simulink model "P_decouple_cascade_rov"  (Simulink 6.0)
settings: Solver=ode45  StartTime=0.0  StopTime=650  RelTol=1e-3
undefined symbols (not defined in the file): B, DQ, DQL, I, m, M, Ma, MaL, MaU, rg, sigbuilder_block, T, W, xb, xg, Xudot, yb, yg, Yvdot, zb, zg, Zwdot
libraries: simulink_extras x27, simulink x20
(part 2 of 5)

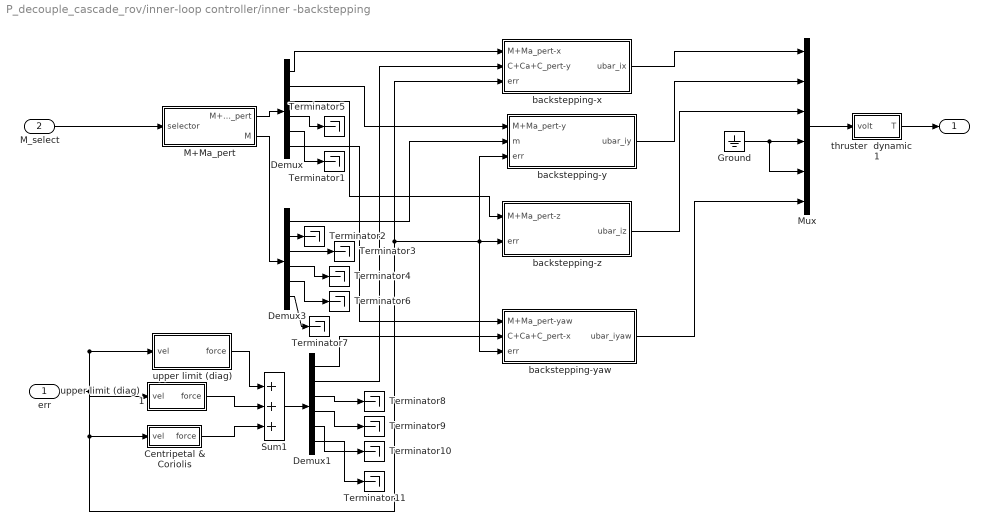
== system P_decouple_cascade_rov/inner-loop controller/inner -backstepping ==
  err : Inport  Port=1  LatchInput=off
  M_select : Inport  Port=2  LatchInput=off
  Centripetal & Coriolis : Subsystem  AncestorBlock=rov_design_analysis/ROV Models/1. Six DOF RRC ROV II/Centripetal & Coriolis
      mask Display: disp('C')
  Demux : Demux  Outputs=6
  Demux1 : Demux  Outputs=6
  Demux3 : Demux  Outputs=6
  Ground : Ground
  M+Ma_pert : Subsystem
  Mux : Mux  Inputs=6
  Sum1 : Sum  Inputs=+++  SaturateOnIntegerOverflow=on  InputSameDT=on
  Terminator{1..11} (11 alike) : Terminator
  backstepping-x : Subsystem
  backstepping-y : Subsystem
  backstepping-yaw : Subsystem
  backstepping-z : Subsystem
  thruster  dynamic     1 : Subsystem
  "upper limit (diag)   " : Subsystem
      mask Display: disp('Perturb CA')
  upper limit (diag)   1 : Subsystem
      mask Display: disp('CA')
  " " : Outport
  wires:
  M_select/1 -> M+Ma_pert/1(selector)
  err/1 -> "upper limit (diag)   "/1(vel), upper limit (diag)   1/1(vel), Centripetal & Coriolis/1(vel), backstepping-x/3(err), backstepping-y/3("err  "), backstepping-z/2("err  "), backstepping-yaw/3(err)
  M+Ma_pert/1(M+Ma_pert) -> Demux/1
  Centripetal & Coriolis/1(force) -> Sum1/3
  upper limit (diag)   1/1(force) -> Sum1/2
  "upper limit (diag)   "/1(force) -> Sum1/1
  Sum1/1 -> Demux1/1
  Demux/1 -> backstepping-x/1(M+Ma_pert-x)
  Demux1/2 -> backstepping-x/2(C+Ca+C_pert-y)
  Mux/1 -> thruster  dynamic     1/1(volt)
  M+Ma_pert/2("M ") -> Demux3/1
  Demux3/1 -> backstepping-y/2(m)
  Demux/2 -> backstepping-y/1(M+Ma_pert-y)
  Demux/6 -> backstepping-yaw/1(M+Ma_pert-yaw)
  Demux1/1 -> backstepping-yaw/2(C+Ca+C_pert-x)
  Demux/3 -> backstepping-z/1(M+Ma_pert-z)
  backstepping-x/1(ubar_ix) -> Mux/1
  backstepping-y/1(ubar_iy) -> Mux/2
  backstepping-z/1(ubar_iz) -> Mux/3
  backstepping-yaw/1(ubar_iyaw) -> Mux/6
  Ground/1 -> Mux/4, Mux/5
  Demux/4 -> Terminator5/1
  Demux/5 -> Terminator1/1
  Demux3/2 -> Terminator2/1
  Demux3/3 -> Terminator3/1
  Demux3/4 -> Terminator4/1
  Demux3/5 -> Terminator6/1
  Demux3/6 -> Terminator7/1
  Demux1/3 -> Terminator8/1
  Demux1/4 -> Terminator9/1
  Demux1/5 -> Terminator10/1
  Demux1/6 -> Terminator11/1
  thruster  dynamic     1/1(T) -> " "/1

== system P_decouple_cascade_rov/inner-loop controller/inner-P ==
  P : Inport  Port=1  LatchInput=off
  Demux1 : Demux
  Ground : Ground
  Mux2 : Mux  Inputs=6
  P Controller{1..4} (4 alike) : simulink_extras/Additional Linear/PID Controller  P=1  I=0  D=0
  Selector : Selector  Elements=[1 2 3 6]  InputPortWidth=6
  thruster  dynamic     1 : Subsystem
  " " : Outport
  wires:
  P Controller3/1 -> Mux2/3
  P Controller1/1 -> Mux2/1
  P Controller2/1 -> Mux2/2
  Selector/1 -> Demux1/1
  Demux1/1 -> P Controller1/1
  Demux1/2 -> P Controller2/1
  Demux1/3 -> P Controller3/1
  Demux1/4 -> P Controller4/1
  P Controller4/1 -> Mux2/6
  Ground/1 -> Mux2/4, Mux2/5
  P/1 -> Selector/1
  Mux2/1 -> thruster  dynamic     1/1(volt)
  thruster  dynamic     1/1(T) -> " "/1

== system P_decouple_cascade_rov/inner-loop controller/inner-sliding ==
  sliding : Inport  Port=1  LatchInput=off
  Sign : Signum
  thruster  dynamic     1 : Subsystem
  " " : Outport
  wires:
  Sign/1 -> thruster  dynamic     1/1(volt)
  sliding/1 -> Sign/1
  thruster  dynamic     1/1(T) -> " "/1

== system P_decouple_cascade_rov/outer-loop  controller/P ==
  err : Inport  Port=1  LatchInput=off
  Demux1 : Demux  Outputs=6
  Mux2 : Mux  Inputs=6
  P Controller{1..4} (4 alike) : simulink_extras/Additional Linear/PID Controller  P=1  I=0  D=0
  " " : Outport
  wires:
  P Controller3/1 -> Mux2/3
  err/1 -> Demux1/1
  Mux2/1 -> " "/1
  Demux1/1 -> P Controller1/1
  P Controller1/1 -> Mux2/1
  P Controller2/1 -> Mux2/2
  P Controller4/1 -> Mux2/6
  Demux1/2 -> P Controller2/1
  Demux1/3 -> P Controller3/1
  Demux1/6 -> P Controller4/1

== system P_decouple_cascade_rov/outer-loop  controller/PI sine +nonlinear  ==
  err : Inport  Port=1  LatchInput=off
  Demux1 : Demux  Outputs=6
  Mux2 : Mux  Inputs=6
  P Controller1 : simulink_extras/Additional Linear/PID Controller  P=1  I=1  D=0
  P Controller2 : simulink_extras/Additional Linear/PID Controller  P=1  I=1  D=0
  P Controller3 : simulink_extras/Additional Linear/PID Controller  P=1  I=1  D=0
  Subsystem : Subsystem
  " " : Outport
  wires:
  P Controller3/1 -> Mux2/3
  err/1 -> Demux1/1
  Mux2/1 -> " "/1
  Demux1/1 -> Subsystem/1(xe), P Controller1/1
  P Controller1/1 -> Mux2/1
  P Controller2/1 -> Mux2/2
  Subsystem/1(yaw_angle) -> Mux2/6
  Demux1/2 -> P Controller2/1, Subsystem/2(ye)
  Demux1/3 -> P Controller3/1

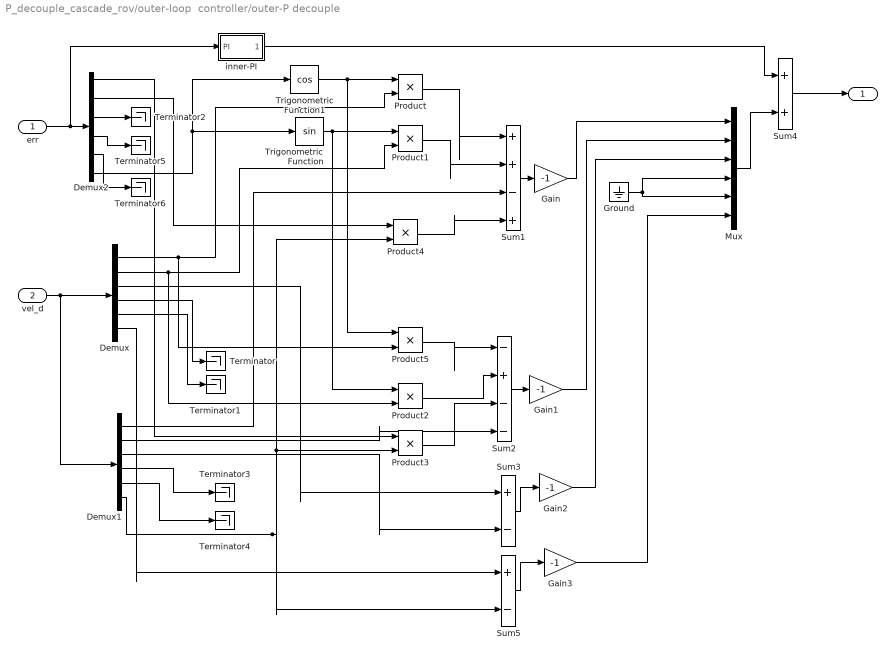
== system P_decouple_cascade_rov/outer-loop  controller/outer-P decouple  ==
  err : Inport  Port=1  LatchInput=off
  vel_d : Inport  Port=2  LatchInput=off
  Demux : Demux  Outputs=6
  Demux1 : Demux  Outputs=6
  Demux2 : Demux  Outputs=6
  Gain{,1..3} (4 alike) : Gain  Gain=-1
  Ground : Ground
  Mux : Mux  Inputs=6
  Product{,1..4} (5 alike) : Product  RndMeth=Zero
  Product5 : Product  OutDataTypeMode=double  RndMeth=Zero
  Sum1 : Sum  Inputs=|++-+  SaturateOnIntegerOverflow=on  InputSameDT=on
  Sum2 : Sum  Inputs=|-+--  SaturateOnIntegerOverflow=on  InputSameDT=on
  Sum3 : Sum  Inputs=|+-  SaturateOnIntegerOverflow=on  InputSameDT=on
  Sum4 : Sum  Inputs=|++  SaturateOnIntegerOverflow=on  InputSameDT=on
  Sum5 : Sum  Inputs=|+-  SaturateOnIntegerOverflow=on  InputSameDT=on
  Terminator{,1..6} (7 alike) : Terminator
  Trigonometric Function : Trigonometry
  Trigonometric Function1 : Trigonometry  Operator=cos
  inner-PI : Subsystem
  " " : Outport
  wires:
  err/1 -> Demux2/1, inner-PI/1(PI)
  vel_d/1 -> Demux/1, Demux1/1
  Sum2/1 -> Gain1/1
  Sum1/1 -> Gain/1
  Sum3/1 -> Gain2/1
  Ground/1 -> Mux/4, Mux/5
  Demux1/4 -> Terminator3/1
  Demux1/5 -> Terminator4/1
  Trigonometric Function/1 -> Product1/1, Product2/1
  Trigonometric Function1/1 -> Product/1, Product5/1
  Demux2/6 -> Trigonometric Function1/1, Trigonometric Function/1
  Demux/1 -> Product5/2, Product/2
  Demux/2 -> Product2/2, Product1/2
  Product/1 -> Sum1/1
  Product1/1 -> Sum1/2
  Demux1/1 -> Sum1/3
  Product4/1 -> Sum1/4
  Demux1/6 -> Product4/2, Product3/2, Sum5/2
  Demux2/2 -> Product4/1
  Product5/1 -> Sum2/1
  Product2/1 -> Sum2/2
  Product3/1 -> Sum2/3
  Demux2/1 -> Product3/1
  Demux1/2 -> Sum2/4
  Demux/3 -> Sum3/1
  Demux1/3 -> Sum3/2
  Demux/4 -> Terminator/1
  Demux/5 -> Terminator1/1
  Gain/1 -> Mux/1
  Gain1/1 -> Mux/2
  Gain2/1 -> Mux/3
  inner-PI/1(" ") -> Sum4/1
  Mux/1 -> Sum4/2
  Sum4/1 -> " "/1
  Demux2/3 -> Terminator2/1
  Demux2/4 -> Terminator5/1
  Demux2/5 -> Terminator6/1
  Demux/6 -> Sum5/1
  Sum5/1 -> Gain3/1
  Gain3/1 -> Mux/6

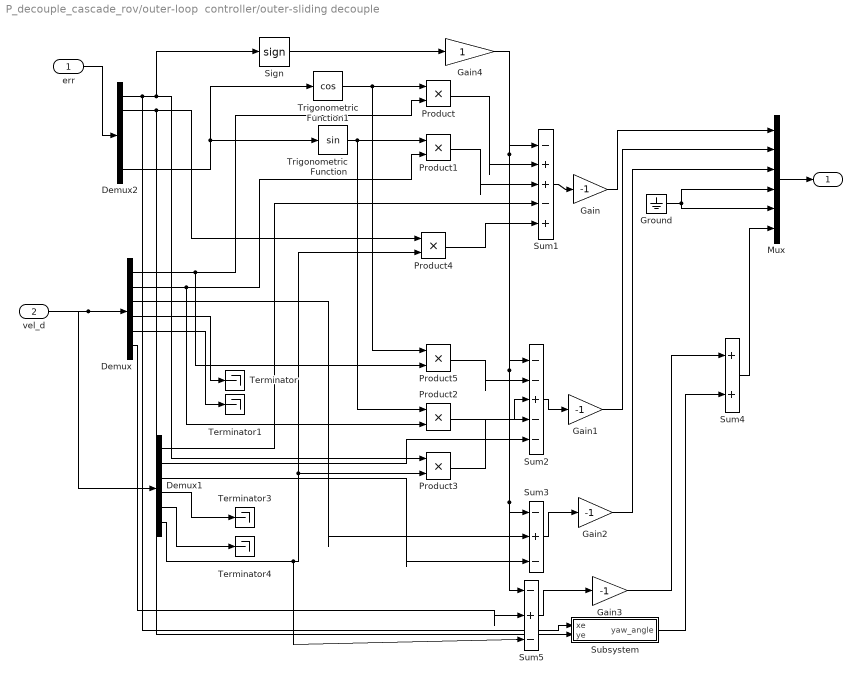
== system P_decouple_cascade_rov/outer-loop  controller/outer-sliding decouple ==
  err : Inport  Port=1  LatchInput=off
  vel_d : Inport  Port=2  LatchInput=off
  Demux : Demux  Outputs=6
  Demux1 : Demux  Outputs=6
  Demux2 : Demux  Outputs=6
  Gain{,1..3} (4 alike) : Gain  Gain=-1
  Gain4 : Gain  SaturateOnIntegerOverflow=on
  Ground : Ground
  Mux : Mux  Inputs=6
  Product{,1..4} (5 alike) : Product  RndMeth=Zero
  Product5 : Product  OutDataTypeMode=double  RndMeth=Zero
  Sign : Signum
  Subsystem : Subsystem
  Sum1 : Sum  Inputs=|-++-+  SaturateOnIntegerOverflow=on  InputSameDT=on
  Sum2 : Sum  Inputs=|--+--  SaturateOnIntegerOverflow=on  InputSameDT=on
  Sum3 : Sum  Inputs=|-+-  SaturateOnIntegerOverflow=on  InputSameDT=on
  Sum4 : Sum  Inputs=|++  SaturateOnIntegerOverflow=on  InputSameDT=on
  Sum5 : Sum  Inputs=|-+-  SaturateOnIntegerOverflow=on  InputSameDT=on
  Terminator{,1,3..4} (4 alike) : Terminator
  Trigonometric Function : Trigonometry
  Trigonometric Function1 : Trigonometry  Operator=cos
  " " : Outport
  wires:
  err/1 -> Demux2/1
  vel_d/1 -> Demux/1, Demux1/1
  Sum2/1 -> Gain1/1
  Sum1/1 -> Gain/1
  Sum3/1 -> Gain2/1
  Sum5/1 -> Gain3/1
  Ground/1 -> Mux/4, Mux/5
  Demux1/4 -> Terminator3/1
  Demux1/5 -> Terminator4/1
  Trigonometric Function/1 -> Product1/1, Product2/1
  Trigonometric Function1/1 -> Product/1, Product5/1
  Demux2/6 -> Trigonometric Function1/1, Trigonometric Function/1
  Demux/1 -> Product/2, Product5/2
  Demux/2 -> Product1/2, Product2/2
  Product/1 -> Sum1/2
  Product1/1 -> Sum1/3
  Demux1/1 -> Sum1/4
  Product4/1 -> Sum1/5
  Demux1/6 -> Product4/2, Product3/2, Sum5/3
  Demux2/2 -> Product4/1, Subsystem/2(ye)
  Product5/1 -> Sum2/2
  Product2/1 -> Sum2/3
  Product3/1 -> Sum2/4
  Demux2/1 -> Product3/1, Sign/1, Subsystem/1(xe)
  Demux1/2 -> Sum2/5
  Demux/3 -> Sum3/2
  Demux1/3 -> Sum3/3
  Demux/6 -> Sum5/2
  Demux/4 -> Terminator/1
  Demux/5 -> Terminator1/1
  Gain/1 -> Mux/1
  Gain1/1 -> Mux/2
  Gain2/1 -> Mux/3
  Sign/1 -> Gain4/1
  Mux/1 -> " "/1
  Gain4/1 -> Sum1/1, Sum2/1, Sum3/1, Sum5/1
  Gain3/1 -> Sum4/1
  Subsystem/1(yaw_angle) -> Sum4/2
  Sum4/1 -> Mux/6

== system P_decouple_cascade_rov/pipeline  tracking planner  /decoupled input ==
  In1 : Inport  Orientation=down  Port=1  LatchInput=off
  relative pt : MultiPortSwitch  Inputs=8
  "x25, y=0, z=50 yaw=1.57" : Subsystem
  "x=0,y=0, z=0 yaw=0  " : Subsystem
  "x=15,y=0, z=45 yaw=0 " : Subsystem
  "x=25, z=45 yaw=0" : Subsystem
  "x=25,y=0, z=50 yaw=0" : Subsystem
  "x=25,y=40, z=50 yaw=0" : Subsystem
  "x=y=0, z=-50 yaw=0  " : Subsystem
  "x=y=15, z=50 yaw=0 " : Subsystem
  Out1 : Outport
  wires:
  "x=y=0, z=-50 yaw=0  "/1("1 ") -> relative pt/2  "1"
  "x=y=15, z=50 yaw=0 "/1(2) -> relative pt/3  "2"
  "x=15,y=0, z=45 yaw=0 "/1(3) -> relative pt/4  "3"
  "x=25, z=45 yaw=0"/1(4) -> relative pt/5  "4"
  "x=25,y=0, z=50 yaw=0"/1(5) -> relative pt/6  "5"
  "x25, y=0, z=50 yaw=1.57"/1(6) -> relative pt/7  "6"
  "x=25,y=40, z=50 yaw=0"/1(7) -> relative pt/8  "7"
  "x=0,y=0, z=0 yaw=0  "/1(8) -> relative pt/9  "8"
  In1/1 -> relative pt/1
  relative pt/1 -> Out1/1

== system P_decouple_cascade_rov/(Observer/ Six DOF RRC ROV   1/Centripetal & Coriolis ==
  vel : Inport  Orientation=up  Port=1  LatchInput=off
  Demux : Demux  Orientation=up  Outputs=2
  Mux : Mux  Inputs=2
  Product{1..5} (5 alike) : Product  SaturateOnIntegerOverflow=on  RndMeth=Zero  InputSameDT=on
  Rg : Constant  Value=rg
  Sum : Sum  SaturateOnIntegerOverflow=on  InputSameDT=on
  Sum1 : Sum  SaturateOnIntegerOverflow=on  InputSameDT=on
  inertia(3x3) : Gain  Gain=I*eye(3)+[Xudot 0 0;0 Yvdot 0;0 0 Zwdot]  Multiplication=Matrix(K*u)  SaturateOnIntegerOverflow=on
  "mass(3x3) " : Gain  Gain=m*eye(3)+[Xudot 0 0;0 Yvdot 0;0 0 Zwdot]  Multiplication=Matrix(K*u)  SaturateOnIntegerOverflow=on
  "mass(3x3)   " : Gain  Gain=m*eye(3)+[Xudot 0 0;0 Yvdot 0;0 0 Zwdot]  Multiplication=Matrix(K*u)  SaturateOnIntegerOverflow=on
  force : Outport  InitialOutput=0
  wires:
  Product1/1 -> Sum/2
  "mass(3x3)   "/1 -> Product2/1
  Product2/1 -> Sum/1
  Rg/1 -> Product3/2, "mass(3x3)   "/1
  Product3/1 -> Product4/2
  Product4/1 -> Sum1/1
  Product5/1 -> Product2/2, Sum1/2
  Sum1/1 -> "mass(3x3) "/1
  Demux/2 -> Product5/1, Product3/1, Product4/1, Product1/1, inertia(3x3)/1
  Demux/1 -> Product5/2
  vel/1 -> Demux/1
  inertia(3x3)/1 -> Product1/2
  "mass(3x3) "/1 -> Mux/1
  Sum/1 -> Mux/2
  Mux/1 -> force/1

== system P_decouple_cascade_rov/(Observer/ Six DOF RRC ROV   1/Hydrodynamic  Damping ==
  vel : Inport  Port=1  LatchInput=off
  D linear : Gain  Gain=-diag(DQL)  SaturateOnIntegerOverflow=on
  damping force : Outport  InitialOutput=0
  wires:
  vel/1 -> D linear/1
  D linear/1 -> damping force/1

== system P_decouple_cascade_rov/(Observer/ Six DOF RRC ROV   1/Hydrodynamic  Damping1 ==
  vel : Inport  Port=1  LatchInput=off
  D quadratic : Gain  Gain=-diag(DQ)  SaturateOnIntegerOverflow=on
  Product : Product  SaturateOnIntegerOverflow=on  RndMeth=Zero  InputSameDT=on
  |u| : Abs  SaturateOnIntegerOverflow=on
  damping force : Outport  InitialOutput=0
  wires:
  Product/1 -> D quadratic/1
  vel/1 -> Product/1, |u|/1
  |u|/1 -> Product/2
  D quadratic/1 -> damping force/1

== system P_decouple_cascade_rov/(Observer/ Six DOF RRC ROV   1/Hydrodynamic  Damping2 ==
  vel : Inport  Port=1  LatchInput=off
  D quadratic : Gain  Gain=0  SaturateOnIntegerOverflow=on
  damping force : Outport  InitialOutput=0
  wires:
  D quadratic/1 -> damping force/1
  vel/1 -> D quadratic/1

== system P_decouple_cascade_rov/(Observer/ Six DOF RRC ROV   1/Mass Inertia Matrix ==
  In : Inport  Port=1  LatchInput=off
  inverse M : Gain  Gain=inv(M-Ma)  Multiplication=Matrix(K*u)  SaturateOnIntegerOverflow=on
  Out : Outport
  wires:
  inverse M/1 -> Out/1
  In/1 -> inverse M/1

== system P_decouple_cascade_rov/(Observer/ Six DOF RRC ROV   1/Restoring Forces ==
  pos : Inport  Port=1  LatchInput=off
  (xg.W-xb.B)cY.cX : Fcn  Expr=(xg*W - xb*B)*cos(u[2])*cos(u[1])
  (zg.W - zb.B)cY.sX : Fcn  Expr=((zg * W - zb * B) * cos(u[2])) * sin(u[1])
  (zg.W - zb.B)sY : Fcn  Expr=(zg*W - zb*B)*sin(u[2])
  -(xg.W-xb.B)cY.sX : Fcn  Expr=-(xg*W - xb*B)*cos(u[2])*sin(u[1])
  -(yg.W-yb.B)cY.cX : Fcn  Expr=-(yg*W - yb*B)*cos(u[2])*cos(u[1])
  -(yg.W-yb.B)sY : Fcn  Expr=-(yg*W - yb*B)*sin(u[2])
  -cY.cX : Fcn  Expr=-cos(u[2])*cos(u[1])
  -cY.sX : Fcn  Expr=-cos(u[2])*sin(u[1])
  Demux : Demux  Outputs=2
  Gain : Gain  Gain=W-B  SaturateOnIntegerOverflow=on
  Mux : Mux  Inputs=3
  Mux1 : Mux
  Sum : Sum  SaturateOnIntegerOverflow=on  InputSameDT=on
  Sum1 : Sum  SaturateOnIntegerOverflow=on  InputSameDT=on
  Sum2 : Sum  SaturateOnIntegerOverflow=on  InputSameDT=on
  Terminator : Terminator
  sY : Fcn  Expr=sin(u[2])
  gravitational force : Outport  InitialOutput=0
  wires:
  Sum2/1 -> Mux1/4
  -(yg.W-yb.B)sY/1 -> Sum2/1
  -(xg.W-xb.B)cY.sX/1 -> Sum2/2
  Sum1/1 -> Mux1/3
  (xg.W-xb.B)cY.cX/1 -> Sum1/1
  (zg.W - zb.B)sY/1 -> Sum1/2
  Sum/1 -> Mux1/2
  (zg.W - zb.B)cY.sX/1 -> Sum/1
  -(yg.W-yb.B)cY.cX/1 -> Sum/2
  Gain/1 -> Mux1/1
  Mux/1 -> Gain/1
  -cY.cX/1 -> Mux/3
  -cY.sX/1 -> Mux/2
  sY/1 -> Mux/1
  Mux1/1 -> gravitational force/1
  Demux/2 -> -(xg.W-xb.B)cY.sX/1, -(yg.W-yb.B)sY/1, (zg.W - zb.B)sY/1, (xg.W-xb.B)cY.cX/1, -(yg.W-yb.B)cY.cX/1, (zg.W - zb.B)cY.sX/1, sY/1, -cY.sX/1, -cY.cX/1
  Demux/1 -> Terminator/1
  pos/1 -> Demux/1

== system P_decouple_cascade_rov/(Observer/ Six DOF RRC ROV   1/lower limit (diag) ==
  In : Inport  Port=1  LatchInput=off
  inverse M : Gain  Gain=-diag([21.1403-21.0981 51.7012-51.0026 92.451-91.837 3.6191-3.576 2.6427-2.7687 2.3033-2.3493])  Multiplication=Matrix(K*u)  SaturateOnIntegerOverflow=on
  Out : Outport
  wires:
  inverse M/1 -> Out/1
  In/1 -> inverse M/1

== system P_decouple_cascade_rov/(Observer/ Six DOF RRC ROV   1/upper limit (diag) ==
  In : Inport  Port=1  LatchInput=off
  inverse M : Gain  Gain=-diag([21.724-21.1403 51.7013-51.7012 94.3-92.451 4.2176-3.6191 7.1148-2.6427 4.7673-2.3033])  Multiplication=Matrix(K*u)  SaturateOnIntegerOverflow=on
  Out : Outport
  wires:
  inverse M/1 -> Out/1
  In/1 -> inverse M/1

== system P_decouple_cascade_rov/(Observer/ Six DOF RRC ROV   1/upper limit (diag)    ==
  note: 7 8 9 10 11 12
  note: 1 2 3 4 5 6
  vel : Inport  Port=1  LatchInput=off
  (zg.W - zb.B)cY.sX : Fcn  Expr=-u[9]*u[3]*u[5]+u[8]*u[2]*u[6]
  (zg.W - zb.B)cY.sX1 : Fcn  Expr=u[9]*u[3]*u[4]-u[7]*u[1]*u[6]
  (zg.W - zb.B)cY.sX2 : Fcn  Expr=-u[8]*u[2]*u[4]+u[7]*u[1]*u[5]
  (zg.W - zb.B)cY.sX3 : Fcn  Expr=-u[9]*u[3]*u[2]+u[8]*u[2]*u[3]-u[12]*u[6]*u[5]+u[11]*u[5]*u[6]
  (zg.W - zb.B)cY.sX4 : Fcn  Expr=u[9]*u[3]*u[1]-u[7]*u[1]*u[3]+u[6]*u[12]*u[4]-u[4]*u[10]*u[6]
  (zg.W - zb.B)cY.sX5 : Fcn  Expr=-u[8]*u[2]*u[1]+u[7]*u[1]*u[2]-u[11]*u[5]*u[4]+u[10]*u[4]*u[5]
  Mux1 : Mux  Inputs=6
  Mux3 : Mux  Inputs=2
  Rg1 : Constant  Value="[MaU(1)  MaU(2)  MaU(3)  MaU(4)  MaU(5)  MaU(6) ]'"
  force : Outport
  wires:
  Mux1/1 -> force/1
  (zg.W - zb.B)cY.sX/1 -> Mux1/1
  (zg.W - zb.B)cY.sX1/1 -> Mux1/2
  (zg.W - zb.B)cY.sX2/1 -> Mux1/3
  (zg.W - zb.B)cY.sX3/1 -> Mux1/4
  (zg.W - zb.B)cY.sX4/1 -> Mux1/5
  (zg.W - zb.B)cY.sX5/1 -> Mux1/6
  vel/1 -> Mux3/1
  Rg1/1 -> Mux3/2
  Mux3/1 -> (zg.W - zb.B)cY.sX/1, (zg.W - zb.B)cY.sX1/1, (zg.W - zb.B)cY.sX4/1, (zg.W - zb.B)cY.sX5/1, (zg.W - zb.B)cY.sX3/1, (zg.W - zb.B)cY.sX2/1

== system P_decouple_cascade_rov/(Observer/ Six DOF RRC ROV   1/upper limit (diag)   1 ==
  note: 7 8 9 10 11 12
  note: 1 2 3 4 5 6
  vel : Inport  Port=1  LatchInput=off
  (zg.W - zb.B)cY.sX : Fcn  Expr=-u[9]*u[3]*u[5]+u[8]*u[2]*u[6]
  (zg.W - zb.B)cY.sX1 : Fcn  Expr=u[9]*u[3]*u[4]-u[7]*u[1]*u[6]
  (zg.W - zb.B)cY.sX2 : Fcn  Expr=-u[8]*u[2]*u[4]+u[7]*u[1]*u[5]
  (zg.W - zb.B)cY.sX3 : Fcn  Expr=-u[9]*u[3]*u[2]+u[8]*u[2]*u[3]-u[12]*u[6]*u[5]+u[11]*u[5]*u[6]
  (zg.W - zb.B)cY.sX4 : Fcn  Expr=u[9]*u[3]*u[1]-u[7]*u[1]*u[3]+u[6]*u[12]*u[4]-u[4]*u[10]*u[6]
  (zg.W - zb.B)cY.sX5 : Fcn  Expr=-u[8]*u[2]*u[1]+u[7]*u[1]*u[2]-u[11]*u[5]*u[4]+u[10]*u[4]*u[5]
  Mux1 : Mux  Inputs=6
  Mux3 : Mux  Inputs=2
  Rg1 : Constant  Value="[Ma(1)  Ma(2)  Ma(3)  Ma(4)  Ma(5)  Ma(6) ]'"
  force : Outport
  wires:
  Mux1/1 -> force/1
  (zg.W - zb.B)cY.sX/1 -> Mux1/1
  (zg.W - zb.B)cY.sX1/1 -> Mux1/2
  (zg.W - zb.B)cY.sX2/1 -> Mux1/3
  (zg.W - zb.B)cY.sX3/1 -> Mux1/4
  (zg.W - zb.B)cY.sX4/1 -> Mux1/5
  (zg.W - zb.B)cY.sX5/1 -> Mux1/6
  vel/1 -> Mux3/1
  Rg1/1 -> Mux3/2
  Mux3/1 -> (zg.W - zb.B)cY.sX/1, (zg.W - zb.B)cY.sX1/1, (zg.W - zb.B)cY.sX4/1, (zg.W - zb.B)cY.sX5/1, (zg.W - zb.B)cY.sX3/1, (zg.W - zb.B)cY.sX2/1

== system P_decouple_cascade_rov/(Observer/ Six DOF RRC ROV   1/upper limit1 ==
  In : Inport  Port=1  LatchInput=off
  inverse M : Gain  Gain=0  Multiplication=Matrix(K*u)  SaturateOnIntegerOverflow=on
  Out : Outport
  wires:
  inverse M/1 -> Out/1
  In/1 -> inverse M/1

== system P_decouple_cascade_rov/(Observer/Euler  Transformation1/Transformation matrix R ==
  angular body  velocity : Inport  Port=1  LatchInput=off
  angular position : Inport  Port=2  LatchInput=off
  Mux : Mux  Inputs=3
  Row1 of T : Subsystem
      mask Display: disp('Row 1')
  Row2 of T : Subsystem
      mask Display: disp('Row 2')
  Row3 of T : Subsystem
      mask Display: disp('Row 3')
  angular earth velocity : Outport
  wires:
  angular position/1 -> Row3 of T/2(angular position), Row1 of T/2(angular position), Row2 of T/2(angular position)
  Mux/1 -> angular earth velocity/1
  Row3 of T/1(angular earth velocity (row 3)) -> Mux/3
  Row2 of T/1(angular earth velocity (row 2)) -> Mux/2
  Row1 of T/1(angular earth velocity (row 1)) -> Mux/1
  angular body  velocity/1 -> Row3 of T/1("angular body velocity "), Row2 of T/1("angular body velocity "), Row1 of T/1(angular body  velocity)

== system P_decouple_cascade_rov/(Observer/Euler  Transformation1/Transformation matrix T ==
  translational body velocity : Inport  Port=1  LatchInput=off
  angular position : Inport  Port=2  LatchInput=off
  Mux : Mux  Inputs=3
  Row1 of R : Subsystem
      mask Display: disp('Row 1')
  Row2 of R : Subsystem
      mask Display: disp('Row 2')
  Row3 of R : Subsystem
      mask Display: disp('Row 3')
  translational earth velocity : Outport  InitialOutput=0
  wires:
  Mux/1 -> translational earth velocity/1
  Row3 of R/1(translational earth velocity (row 3)) -> Mux/3
  Row2 of R/1(translational earth velocity (row 2)) -> Mux/2
  Row1 of R/1(translational earth velocity (row 1)) -> Mux/1
  angular position/1 -> Row3 of R/2(angular position), Row1 of R/2(angular position), Row2 of R/2(angular position)
  translational body velocity/1 -> Row1 of R/1(translational body velocity), Row2 of R/1(translational body velocity), Row3 of R/1(translational body velocity)

== system P_decouple_cascade_rov/(Observer/Thruster  Dynamic/Thruster configuration1 ==
  input velocity : Inport  Orientation=up  Port=1  LatchInput=off
  Thruster Matrix : Gain  Gain=T  Multiplication=Matrix(K*u)  SaturateOnIntegerOverflow=on
  output force : Outport  InitialOutput=0
  wires:
  input velocity/1 -> Thruster Matrix/1
  Thruster Matrix/1 -> output force/1

== system P_decouple_cascade_rov/(Observer/Thruster  Dynamic/Thruster configuration4 ==
  input velocity : Inport  Orientation=up  Port=1  LatchInput=off
  Thruster Matrix : Gain  Gain=T  Multiplication=Matrix(K*u)  SaturateOnIntegerOverflow=on
  output force : Outport  InitialOutput=0
  wires:
  input velocity/1 -> Thruster Matrix/1
  Thruster Matrix/1 -> output force/1

== system P_decouple_cascade_rov/(Observer/Thruster  Dynamic/thruster  dynamic     1 ==
  volt : Inport  Orientation=down  Port=1  LatchInput=off
  Gain2 : Gain  Gain=0.5  SaturateOnIntegerOverflow=on
  Saturation : Saturate  UpperLimit=70  LowerLimit=-70
  "thruster  alloc. " : Subsystem
  T : Outport
  wires:
  volt/1 -> "thruster  alloc. "/1(err)
  "thruster  alloc. "/1(u) -> Gain2/1
  Saturation/1 -> T/1
  Gain2/1 -> Saturation/1

== system P_decouple_cascade_rov/(Observer/inner-loop controller1/inner -PI-decouple  ==
  err : Inport  Port=1  LatchInput=off
  Centripetal & Coriolis : Subsystem  AncestorBlock=rov_design_analysis/ROV Models/1. Six DOF RRC ROV II/Centripetal & Coriolis
      mask Display: disp('C')
  Gain2 : Gain  SaturateOnIntegerOverflow=on
  Hydrodynamic  Damping : Subsystem
      mask Display: disp('D')
  Hydrodynamic  Damping1 : Subsystem
      mask Display: disp('Perturb D')
  Sum : Sum  Inputs=|-++  SaturateOnIntegerOverflow=on  InputSameDT=on
  Sum1 : Sum  Inputs=+++  SaturateOnIntegerOverflow=on  InputSameDT=on
  Sum5 : Sum  Inputs=|++  SaturateOnIntegerOverflow=on  InputSameDT=on
  inner-PI : Subsystem
  thruster  dynamic     1 : Subsystem
  "upper limit (diag)   " : Subsystem
      mask Display: disp('Perturb CA')
  upper limit (diag)   1 : Subsystem
      mask Display: disp('CA')
  " " : Outport
  wires:
  err/1 -> upper limit (diag)   1/1(vel), Centripetal & Coriolis/1(vel), "upper limit (diag)   "/1(vel), Hydrodynamic  Damping/1(vel), Hydrodynamic  Damping1/1(vel), inner-PI/1(PI)
  upper limit (diag)   1/1(force) -> Sum1/1
  Centripetal & Coriolis/1(force) -> Sum1/2
  Hydrodynamic  Damping1/1(damping force) -> Sum5/2
  inner-PI/1(" ") -> Gain2/1
  "upper limit (diag)   "/1(force) -> Sum1/3
  Hydrodynamic  Damping/1(damping force) -> Sum5/1
  Gain2/1 -> Sum/1
  Sum5/1 -> Sum/3
  Sum1/1 -> Sum/2
  Sum/1 -> thruster  dynamic     1/1(volt)
  thruster  dynamic     1/1(T) -> " "/1

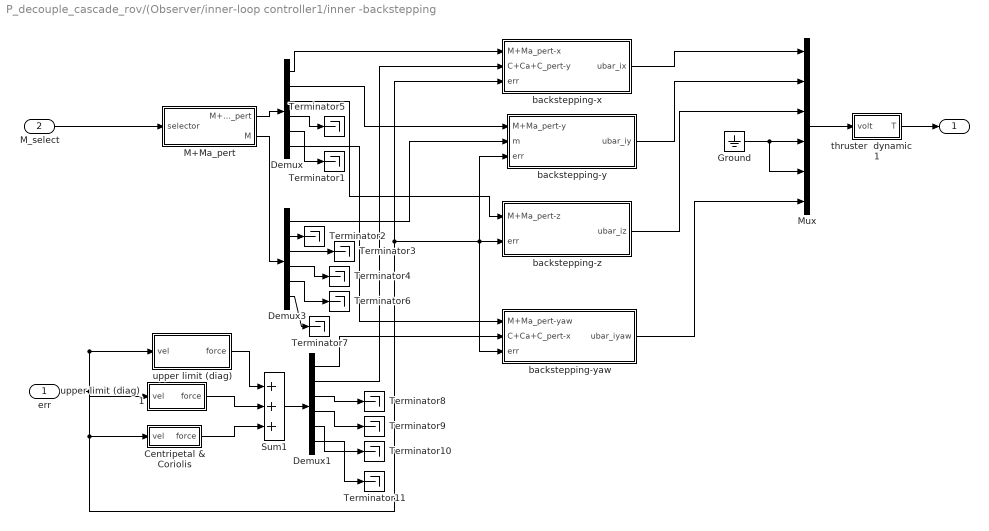
== system P_decouple_cascade_rov/(Observer/inner-loop controller1/inner -backstepping ==
  err : Inport  Port=1  LatchInput=off
  M_select : Inport  Port=2  LatchInput=off
  Centripetal & Coriolis : Subsystem  AncestorBlock=rov_design_analysis/ROV Models/1. Six DOF RRC ROV II/Centripetal & Coriolis
      mask Display: disp('C')
  Demux : Demux  Outputs=6
  Demux1 : Demux  Outputs=6
  Demux3 : Demux  Outputs=6
  Ground : Ground
  M+Ma_pert : Subsystem
  Mux : Mux  Inputs=6
  Sum1 : Sum  Inputs=+++  SaturateOnIntegerOverflow=on  InputSameDT=on
  Terminator{1..11} (11 alike) : Terminator
  backstepping-x : Subsystem
  backstepping-y : Subsystem
  backstepping-yaw : Subsystem
  backstepping-z : Subsystem
  thruster  dynamic     1 : Subsystem
  "upper limit (diag)   " : Subsystem
      mask Display: disp('Perturb CA')
  upper limit (diag)   1 : Subsystem
      mask Display: disp('CA')
  " " : Outport
  wires:
  M_select/1 -> M+Ma_pert/1(selector)
  err/1 -> "upper limit (diag)   "/1(vel), upper limit (diag)   1/1(vel), Centripetal & Coriolis/1(vel), backstepping-x/3(err), backstepping-y/3("err  "), backstepping-z/2("err  "), backstepping-yaw/3(err)
  M+Ma_pert/1(M+Ma_pert) -> Demux/1
  Centripetal & Coriolis/1(force) -> Sum1/3
  upper limit (diag)   1/1(force) -> Sum1/2
  "upper limit (diag)   "/1(force) -> Sum1/1
  Sum1/1 -> Demux1/1
  Demux/1 -> backstepping-x/1(M+Ma_pert-x)
  Demux1/2 -> backstepping-x/2(C+Ca+C_pert-y)
  Mux/1 -> thruster  dynamic     1/1(volt)
  M+Ma_pert/2("M ") -> Demux3/1
  Demux3/1 -> backstepping-y/2(m)
  Demux/2 -> backstepping-y/1(M+Ma_pert-y)
  Demux/6 -> backstepping-yaw/1(M+Ma_pert-yaw)
  Demux1/1 -> backstepping-yaw/2(C+Ca+C_pert-x)
  Demux/3 -> backstepping-z/1(M+Ma_pert-z)
  backstepping-x/1(ubar_ix) -> Mux/1
  backstepping-y/1(ubar_iy) -> Mux/2
  backstepping-z/1(ubar_iz) -> Mux/3
  backstepping-yaw/1(ubar_iyaw) -> Mux/6
  Ground/1 -> Mux/4, Mux/5
  Demux/4 -> Terminator5/1
  Demux/5 -> Terminator1/1
  Demux3/2 -> Terminator2/1
  Demux3/3 -> Terminator3/1
  Demux3/4 -> Terminator4/1
  Demux3/5 -> Terminator6/1
  Demux3/6 -> Terminator7/1
  Demux1/3 -> Terminator8/1
  Demux1/4 -> Terminator9/1
  Demux1/5 -> Terminator10/1
  Demux1/6 -> Terminator11/1
  thruster  dynamic     1/1(T) -> " "/1

== system P_decouple_cascade_rov/(Observer/inner-loop controller1/inner-P ==
  P : Inport  Port=1  LatchInput=off
  Demux1 : Demux
  Ground : Ground
  Mux2 : Mux  Inputs=6
  P Controller{1..4} (4 alike) : simulink_extras/Additional Linear/PID Controller  P=1  I=0  D=0
  Selector : Selector  Elements=[1 2 3 6]  InputPortWidth=6
  thruster  dynamic     1 : Subsystem
  " " : Outport
  wires:
  P Controller3/1 -> Mux2/3
  P Controller1/1 -> Mux2/1
  P Controller2/1 -> Mux2/2
  Selector/1 -> Demux1/1
  Demux1/1 -> P Controller1/1
  Demux1/2 -> P Controller2/1
  Demux1/3 -> P Controller3/1
  Demux1/4 -> P Controller4/1
  P Controller4/1 -> Mux2/6
  Ground/1 -> Mux2/4, Mux2/5
  P/1 -> Selector/1
  Mux2/1 -> thruster  dynamic     1/1(volt)
  thruster  dynamic     1/1(T) -> " "/1

== system P_decouple_cascade_rov/(Observer/inner-loop controller1/inner-sliding ==
  sliding : Inport  Port=1  LatchInput=off
  Sign : Signum
  thruster  dynamic     1 : Subsystem
  " " : Outport
  wires:
  Sign/1 -> thruster  dynamic     1/1(volt)
  sliding/1 -> Sign/1
  thruster  dynamic     1/1(T) -> " "/1

== system P_decouple_cascade_rov/Euler  Transformation/Transformation matrix R/Row1 of T ==
  angular body  velocity : Inport  Port=1  LatchInput=off
  angular position : Inport  Port=2  LatchInput=off
  1 : Fcn  Expr=1
  Dot Product1 : simulink/Math Operations/Dot Product  InputSameDT=on  OutDataType=sfix(16)  OutScaling=2^-10  DoSatur=off
  Mux1 : Mux  Inputs=3
  cX.tY : Fcn  Expr=cos(u[1])*tan(u[2])
  sX.tY : Fcn  Expr=sin(u[1])*tan(u[2])
  angular earth velocity (row 1) : Outport
  wires:
  Dot Product1/1 -> angular earth velocity (row 1)/1
  angular body  velocity/1 -> Dot Product1/2
  Mux1/1 -> Dot Product1/1
  cX.tY/1 -> Mux1/3
  sX.tY/1 -> Mux1/2
  1/1 -> Mux1/1
  angular position/1 -> cX.tY/1, sX.tY/1, 1/1

== system P_decouple_cascade_rov/Euler  Transformation/Transformation matrix R/Row2 of T ==
  "angular body velocity " : Inport  Port=1  LatchInput=off
  angular position : Inport  Port=2  LatchInput=off
  -sX : Fcn  Expr=-sin(u[1])
  0 : Fcn  Expr=0
  Dot Product1 : simulink/Math Operations/Dot Product  InputSameDT=on  OutDataType=sfix(16)  OutScaling=2^-10  DoSatur=off
  Mux1 : Mux  Inputs=3
  cX : Fcn  Expr=cos(u[1])
  angular earth velocity (row 2) : Outport
  wires:
  Dot Product1/1 -> angular earth velocity (row 2)/1
  "angular body velocity "/1 -> Dot Product1/2
  Mux1/1 -> Dot Product1/1
  -sX/1 -> Mux1/3
  cX/1 -> Mux1/2
  0/1 -> Mux1/1
  angular position/1 -> -sX/1, cX/1, 0/1

== system P_decouple_cascade_rov/Euler  Transformation/Transformation matrix R/Row3 of T ==
  "angular body velocity " : Inport  Port=1  LatchInput=off
  angular position : Inport  Port=2  LatchInput=off
  1 : Fcn  Expr=0
  Dot Product1 : simulink/Math Operations/Dot Product  InputSameDT=on  OutDataType=sfix(16)  OutScaling=2^-10  DoSatur=off
  Mux1 : Mux  Inputs=3
  cX/cY : Fcn  Expr=cos(u[1])/cos(u[2])
  sX/cY : Fcn  Expr=sin(u[1])/cos(u[2])
  angular earth velocity (row 3) : Outport
  wires:
  Dot Product1/1 -> angular earth velocity (row 3)/1
  "angular body velocity "/1 -> Dot Product1/2
  Mux1/1 -> Dot Product1/1
  cX/cY/1 -> Mux1/3
  sX/cY/1 -> Mux1/2
  1/1 -> Mux1/1
  angular position/1 -> cX/cY/1, sX/cY/1, 1/1

== system P_decouple_cascade_rov/Euler  Transformation/Transformation matrix T/Row1 of R ==
  translational body velocity : Inport  Port=1  LatchInput=off
  angular position : Inport  Port=2  LatchInput=off
  -sZ.cX+cZ.sY.sX : Fcn  Expr=-sin(u[3])*cos(u[1]) + cos(u[3])*sin(u[2])*sin(u[1])
  Dot Product : simulink/Math Operations/Dot Product  InputSameDT=on  OutDataType=sfix(16)  OutScaling=2^-10  DoSatur=off
  Mux : Mux  Inputs=3
  cY.cZ : Fcn  Expr=cos(u[3]) * cos(u[2])
  sZ.sX+cZ.cX.sY : Fcn  Expr=sin(u[3])*sin(u[1]) + cos(u[3])*cos(u[1])*sin(u[2])
  translational earth velocity (row 1) : Outport
  wires:
  Dot Product/1 -> translational earth velocity (row 1)/1
  translational body velocity/1 -> Dot Product/2
  Mux/1 -> Dot Product/1
  sZ.sX+cZ.cX.sY/1 -> Mux/3
  -sZ.cX+cZ.sY.sX/1 -> Mux/2
  cY.cZ/1 -> Mux/1
  angular position/1 -> sZ.sX+cZ.cX.sY/1, -sZ.cX+cZ.sY.sX/1, cY.cZ/1

== system P_decouple_cascade_rov/Euler  Transformation/Transformation matrix T/Row2 of R ==
  translational body velocity : Inport  Port=1  LatchInput=off
  angular position : Inport  Port=2  LatchInput=off
  -cZ.sX+sY.sZ.cX : Fcn  Expr=-cos(u[3])*sin(u[1]) + sin(u[2])*sin(u[3])*cos(u[1])
  Dot Product1 : simulink/Math Operations/Dot Product  InputSameDT=on  OutDataType=sfix(16)  OutScaling=2^-10  DoSatur=off
  Mux1 : Mux  Inputs=3
  cY.sZ : Fcn  Expr=sin(u[3]) * cos(u[2])
  cZ.cX+sX.sY.sZ : Fcn  Expr=cos(u[3])*cos(u[1]) + sin(u[1])*sin(u[2])*sin(u[3])
  translational earth velocity (row 2) : Outport
  wires:
  Dot Product1/1 -> translational earth velocity (row 2)/1
  translational body velocity/1 -> Dot Product1/2
  Mux1/1 -> Dot Product1/1
  -cZ.sX+sY.sZ.cX/1 -> Mux1/3
  cZ.cX+sX.sY.sZ/1 -> Mux1/2
  cY.sZ/1 -> Mux1/1
  angular position/1 -> -cZ.sX+sY.sZ.cX/1, cZ.cX+sX.sY.sZ/1, cY.sZ/1

== system P_decouple_cascade_rov/Euler  Transformation/Transformation matrix T/Row3 of R ==
  translational body velocity : Inport  Port=1  LatchInput=off
  angular position : Inport  Port=2  LatchInput=off
  -sY : Fcn  Expr=-sin(u[2])
  Dot Product1 : simulink/Math Operations/Dot Product  InputSameDT=on  OutDataType=sfix(16)  OutScaling=2^-10  DoSatur=off
  Mux1 : Mux  Inputs=3
  cY.cX : Fcn  Expr=cos(u[2])*cos(u[1])
  cY.sX : Fcn  Expr=cos(u[2])*sin(u[1])
  translational earth velocity (row 3) : Outport  InitialOutput=0
  wires:
  Dot Product1/1 -> translational earth velocity (row 3)/1
  translational body velocity/1 -> Dot Product1/2
  Mux1/1 -> Dot Product1/1
  cY.cX/1 -> Mux1/3
  cY.sX/1 -> Mux1/2
  -sY/1 -> Mux1/1
  angular position/1 -> cY.cX/1, cY.sX/1, -sY/1

== system P_decouple_cascade_rov/Supervisor (Logic - based)/Switching sequence/Signal Builder2 ==
  Demux : Demux  Tag=STV Demux  Outputs=7
  FromWs : FromWorkspace  Tag=STV FromWs  VariableName=tuvar  SampleTime=0  SigBuilderData=DataTag0  VnvData=DataTag1
      SigBuilderData=|
      | channels(1).label = 'Signal 1'
      | channels(1).allXData = {[0 65 65 700]}
      | channels(1).allYData = {[1 1 0 0]}
      | channels(2).label = 'Signal 2'
      | channels(2).allXData = {[0 70 70 150 150 700]}
      | channels(2).allYData = {[0 0 1 1 0 0]}
      | channels(3).label = 'Signal 3'
      | channels(3).allXData = {[0 160 160 230 230 700]}
      | channels(3).allYData = {[0 0 1 1 0 0]}
      | channels(4).label = 'Signal 4'
      | channels(4).allXData = {[0 240 240 290 290 700]}
      | channels(4).allYData = {[0 0 1 1 0 0]}
      | channels(5).label = 'Signal 5'
      | channels(5).allXData = {[0 300 300 350 350 700]}
      | channels(5).allYData = {[0 0 1 1 0 0]}
      | channels(6).label = 'Signal 6'
      | channels(6).allXData = {[0 360 360 400 400 700]}
      | channels(6).allYData = {[0 0 1 1 0 0]}
      | channels(7).label = 'Signal 7'
      | channels(7).allXData = {[0 410 410 548 548 700]}
      | channels(7).allYData = {[0 0 1 1 0 0]}
      | dataSet.timeRange = [0 700]
      | dataSet.name = 'Group 1'
  Signal 1 : Outport  Tag=STV Outport
  Signal 2 : Outport  Tag=STV Outport  Port=2
  Signal 3 : Outport  Tag=STV Outport  Port=3
  Signal 4 : Outport  Tag=STV Outport  Port=4
  Signal 5 : Outport  Tag=STV Outport  Port=5
  Signal 6 : Outport  Tag=STV Outport  Port=6
  Signal 7 : Outport  Tag=STV Outport  Port=7
  wires:
  Demux/7 -> Signal 7/1
  Demux/6 -> Signal 6/1
  Demux/5 -> Signal 5/1
  Demux/4 -> Signal 4/1
  Demux/3 -> Signal 3/1
  Demux/2 -> Signal 2/1
  FromWs/1 -> Demux/1
  Demux/1 -> Signal 1/1

== system P_decouple_cascade_rov/Supervisor (Logic - based)/Switching sequence1/Signal Builder2 ==
  Demux : Demux  Tag=STV Demux  Outputs=7
  FromWs : FromWorkspace  Tag=STV FromWs  VariableName=tuvar  SampleTime=0  SigBuilderData=DataTag2  VnvData=DataTag3
      SigBuilderData=|
      | channels(1).label = 'Signal 1'
      | channels(1).allXData = {[0 65 65 700]}
      | channels(1).allYData = {[1 1 0 0]}
      | channels(2).label = 'Signal 2'
      | channels(2).allXData = {[0 70 70 150 150 700]}
      | channels(2).allYData = {[0 0 1 1 0 0]}
      | channels(3).label = 'Signal 3'
      | channels(3).allXData = {[0 160 160 230 230 700]}
      | channels(3).allYData = {[0 0 1 1 0 0]}
      | channels(4).label = 'Signal 4'
      | channels(4).allXData = {[0 240 240 290 290 700]}
      | channels(4).allYData = {[0 0 1 1 0 0]}
      | channels(5).label = 'Signal 5'
      | channels(5).allXData = {[0 300 300 350 350 700]}
      | channels(5).allYData = {[0 0 1 1 0 0]}
      | channels(6).label = 'Signal 6'
      | channels(6).allXData = {[0 360 360 400 400 700]}
      | channels(6).allYData = {[0 0 1 1 0 0]}
      | channels(7).label = 'Signal 7'
      | channels(7).allXData = {[0 410 410 548 548 700]}
      | channels(7).allYData = {[0 0 1 1 0 0]}
      | dataSet.timeRange = [0 700]
      | dataSet.name = 'Group 1'
  Signal 1 : Outport  Tag=STV Outport
  Signal 2 : Outport  Tag=STV Outport  Port=2
  Signal 3 : Outport  Tag=STV Outport  Port=3
  Signal 4 : Outport  Tag=STV Outport  Port=4
  Signal 5 : Outport  Tag=STV Outport  Port=5
  Signal 6 : Outport  Tag=STV Outport  Port=6
  Signal 7 : Outport  Tag=STV Outport  Port=7
  wires:
  Demux/7 -> Signal 7/1
  Demux/6 -> Signal 6/1
  Demux/5 -> Signal 5/1
  Demux/4 -> Signal 4/1
  Demux/3 -> Signal 3/1
  Demux/2 -> Signal 2/1
  FromWs/1 -> Demux/1
  Demux/1 -> Signal 1/1

== system P_decouple_cascade_rov/Thruster  Dynamic/thruster  dynamic     1/thruster  alloc.  ==
  err : Inport  Port=1  LatchInput=off
  " input" : Constant  Value=[ 1 1 1 1]'
  Selector : Selector  Elements=[1 2 3 6]  InputPortWidth=6
  thruster  allocation control1 : Subsystem  AncestorBlock=|
      | rov_design_analysis/ROV Controller
      | Design
      | Applications/1. Heading autopilot/thruster 
      | allocation control
  u : Outport
  wires:
  err/1 -> Selector/1
  Selector/1 -> thruster  allocation control1/1(vel)
  " input"/1 -> thruster  allocation control1/2(on/off)
  thruster  allocation control1/1(volt) -> u/1

== system P_decouple_cascade_rov/inner-loop controller/inner -PI-decouple /Centripetal & Coriolis ==
  vel : Inport  Orientation=up  Port=1  LatchInput=off
  Demux : Demux  Orientation=up  Outputs=2
  Mux : Mux  Inputs=2
  Product{1..5} (5 alike) : Product  SaturateOnIntegerOverflow=on  RndMeth=Zero  InputSameDT=on
  Rg : Constant  Value=rg
  Sum : Sum  SaturateOnIntegerOverflow=on  InputSameDT=on
  Sum1 : Sum  SaturateOnIntegerOverflow=on  InputSameDT=on
  inertia(3x3) : Gain  Gain=I  Multiplication=Matrix(K*u)  SaturateOnIntegerOverflow=on
  "mass(3x3) " : Gain  Gain=m  Multiplication=Matrix(K*u)  SaturateOnIntegerOverflow=on
  "mass(3x3)   " : Gain  Gain=m  Multiplication=Matrix(K*u)  SaturateOnIntegerOverflow=on
  force : Outport  InitialOutput=0
  wires:
  Product1/1 -> Sum/2
  "mass(3x3)   "/1 -> Product2/1
  Product2/1 -> Sum/1
  Rg/1 -> Product3/2, "mass(3x3)   "/1
  Product3/1 -> Product4/2
  Product4/1 -> Sum1/1
  Product5/1 -> Product2/2, Sum1/2
  Sum1/1 -> "mass(3x3) "/1
  Demux/2 -> Product5/1, Product3/1, Product4/1, Product1/1, inertia(3x3)/1
  Demux/1 -> Product5/2
  vel/1 -> Demux/1
  inertia(3x3)/1 -> Product1/2
  "mass(3x3) "/1 -> Mux/1
  Sum/1 -> Mux/2
  Mux/1 -> force/1

== system P_decouple_cascade_rov/inner-loop controller/inner -PI-decouple /Hydrodynamic  Damping ==
  vel : Inport  Port=1  LatchInput=off
  D linear : Gain  Gain=-diag(DQL)  SaturateOnIntegerOverflow=on
  damping force : Outport  InitialOutput=0
  wires:
  vel/1 -> D linear/1
  D linear/1 -> damping force/1

== system P_decouple_cascade_rov/inner-loop controller/inner -PI-decouple /Hydrodynamic  Damping1 ==
  vel : Inport  Port=1  LatchInput=off
  D quadratic : Gain  Gain=-diag(DQ)  SaturateOnIntegerOverflow=on
  Product : Product  SaturateOnIntegerOverflow=on  RndMeth=Zero  InputSameDT=on
  |u| : Abs  SaturateOnIntegerOverflow=on
  damping force : Outport  InitialOutput=0
  wires:
  Product/1 -> D quadratic/1
  vel/1 -> Product/1, |u|/1
  |u|/1 -> Product/2
  D quadratic/1 -> damping force/1

== system P_decouple_cascade_rov/inner-loop controller/inner -PI-decouple /inner-PI ==
  PI : Inport  Port=1  LatchInput=off
  Demux1 : Demux
  Ground : Ground
  Mux2 : Mux  Inputs=6
  P Controller{1..4} (4 alike) : simulink_extras/Additional Linear/PID Controller  P=1  I=0  D=0
  Selector : Selector  Elements=[1 2 3 6]  InputPortWidth=6
  " " : Outport
  wires:
  P Controller3/1 -> Mux2/3
  P Controller1/1 -> Mux2/1
  P Controller2/1 -> Mux2/2
  Selector/1 -> Demux1/1
  Demux1/1 -> P Controller1/1
  Demux1/2 -> P Controller2/1
  Demux1/3 -> P Controller3/1
  Demux1/4 -> P Controller4/1
  P Controller4/1 -> Mux2/6
  Ground/1 -> Mux2/4, Mux2/5
  PI/1 -> Selector/1
  Mux2/1 -> " "/1

== system P_decouple_cascade_rov/inner-loop controller/inner -PI-decouple /thruster  dynamic     1 ==
  volt : Inport  Orientation=down  Port=1  LatchInput=off
  Gain2 : Gain  Gain=0.5  SaturateOnIntegerOverflow=on
  Saturation : Saturate  UpperLimit=70  LowerLimit=-70
  "thruster  alloc. " : Subsystem
  T : Outport
  wires:
  volt/1 -> "thruster  alloc. "/1(err)
  "thruster  alloc. "/1(u) -> Gain2/1
  Saturation/1 -> T/1
  Gain2/1 -> Saturation/1

== system P_decouple_cascade_rov/inner-loop controller/inner -PI-decouple /upper limit (diag)    ==
  note: 7 8 9 10 11 12
  note: 1 2 3 4 5 6
  vel : Inport  Port=1  LatchInput=off
  (zg.W - zb.B)cY.sX : Fcn  Expr=-u[9]*u[3]*u[5]+u[8]*u[2]*u[6]
  (zg.W - zb.B)cY.sX1 : Fcn  Expr=u[9]*u[3]*u[4]-u[7]*u[1]*u[6]
  (zg.W - zb.B)cY.sX2 : Fcn  Expr=-u[8]*u[2]*u[4]+u[7]*u[1]*u[5]
  (zg.W - zb.B)cY.sX3 : Fcn  Expr=-u[9]*u[3]*u[2]+u[8]*u[2]*u[3]-u[12]*u[6]*u[5]+u[11]*u[5]*u[6]
  (zg.W - zb.B)cY.sX4 : Fcn  Expr=u[9]*u[3]*u[1]-u[7]*u[1]*u[3]+u[6]*u[12]*u[4]-u[4]*u[10]*u[6]
  (zg.W - zb.B)cY.sX5 : Fcn  Expr=-u[8]*u[2]*u[1]+u[7]*u[1]*u[2]-u[11]*u[5]*u[4]+u[10]*u[4]*u[5]
  Mux1 : Mux  Inputs=6
  Mux3 : Mux  Inputs=2
  Rg2 : Constant  Value="[MaU(1)  MaU(2)  MaU(3)  MaU(4)  MaU(5)  MaU(6) ]'"
  force : Outport
  wires:
  Mux1/1 -> force/1
  (zg.W - zb.B)cY.sX/1 -> Mux1/1
  (zg.W - zb.B)cY.sX1/1 -> Mux1/2
  (zg.W - zb.B)cY.sX2/1 -> Mux1/3
  (zg.W - zb.B)cY.sX3/1 -> Mux1/4
  (zg.W - zb.B)cY.sX4/1 -> Mux1/5
  (zg.W - zb.B)cY.sX5/1 -> Mux1/6
  vel/1 -> Mux3/1
  Rg2/1 -> Mux3/2
  Mux3/1 -> (zg.W - zb.B)cY.sX/1, (zg.W - zb.B)cY.sX1/1, (zg.W - zb.B)cY.sX4/1, (zg.W - zb.B)cY.sX5/1, (zg.W - zb.B)cY.sX3/1, (zg.W - zb.B)cY.sX2/1

== system P_decouple_cascade_rov/inner-loop controller/inner -PI-decouple /upper limit (diag)   1 ==
  note: 7 8 9 10 11 12
  note: 1 2 3 4 5 6
  vel : Inport  Port=1  LatchInput=off
  (zg.W - zb.B)cY.sX : Fcn  Expr=-u[9]*u[3]*u[5]+u[8]*u[2]*u[6]
  (zg.W - zb.B)cY.sX1 : Fcn  Expr=u[9]*u[3]*u[4]-u[7]*u[1]*u[6]
  (zg.W - zb.B)cY.sX2 : Fcn  Expr=-u[8]*u[2]*u[4]+u[7]*u[1]*u[5]
  (zg.W - zb.B)cY.sX3 : Fcn  Expr=-u[9]*u[3]*u[2]+u[8]*u[2]*u[3]-u[12]*u[6]*u[5]+u[11]*u[5]*u[6]
  (zg.W - zb.B)cY.sX4 : Fcn  Expr=u[9]*u[3]*u[1]-u[7]*u[1]*u[3]+u[6]*u[12]*u[4]-u[4]*u[10]*u[6]
  (zg.W - zb.B)cY.sX5 : Fcn  Expr=-u[8]*u[2]*u[1]+u[7]*u[1]*u[2]-u[11]*u[5]*u[4]+u[10]*u[4]*u[5]
  Mux1 : Mux  Inputs=6
  Mux3 : Mux  Inputs=2
  Rg1 : Constant  Value="[Ma(1)  Ma(2)  Ma(3)  Ma(4)  Ma(5)  Ma(6) ]'"
  force : Outport
  wires:
  Mux1/1 -> force/1
  (zg.W - zb.B)cY.sX/1 -> Mux1/1
  (zg.W - zb.B)cY.sX1/1 -> Mux1/2
  (zg.W - zb.B)cY.sX2/1 -> Mux1/3
  (zg.W - zb.B)cY.sX3/1 -> Mux1/4
  (zg.W - zb.B)cY.sX4/1 -> Mux1/5
  (zg.W - zb.B)cY.sX5/1 -> Mux1/6
  vel/1 -> Mux3/1
  Rg1/1 -> Mux3/2
  Mux3/1 -> (zg.W - zb.B)cY.sX/1, (zg.W - zb.B)cY.sX1/1, (zg.W - zb.B)cY.sX4/1, (zg.W - zb.B)cY.sX5/1, (zg.W - zb.B)cY.sX3/1, (zg.W - zb.B)cY.sX2/1

== system P_decouple_cascade_rov/inner-loop controller/inner -backstepping/Centripetal & Coriolis ==
  vel : Inport  Orientation=up  Port=1  LatchInput=off
  Demux : Demux  Orientation=up  Outputs=2
  Mux : Mux  Inputs=2
  Product{1..5} (5 alike) : Product  SaturateOnIntegerOverflow=on  RndMeth=Zero  InputSameDT=on
  Rg : Constant  Value=rg
  Sum : Sum  SaturateOnIntegerOverflow=on  InputSameDT=on
  Sum1 : Sum  SaturateOnIntegerOverflow=on  InputSameDT=on
  inertia(3x3) : Gain  Gain=I  Multiplication=Matrix(K*u)  SaturateOnIntegerOverflow=on
  "mass(3x3) " : Gain  Gain=m  Multiplication=Matrix(K*u)  SaturateOnIntegerOverflow=on
  "mass(3x3)   " : Gain  Gain=m  Multiplication=Matrix(K*u)  SaturateOnIntegerOverflow=on
  force : Outport  InitialOutput=0
  wires:
  Product1/1 -> Sum/2
  "mass(3x3)   "/1 -> Product2/1
  Product2/1 -> Sum/1
  Rg/1 -> Product3/2, "mass(3x3)   "/1
  Product3/1 -> Product4/2
  Product4/1 -> Sum1/1
  Product5/1 -> Product2/2, Sum1/2
  Sum1/1 -> "mass(3x3) "/1
  Demux/2 -> Product5/1, Product3/1, Product4/1, Product1/1, inertia(3x3)/1
  Demux/1 -> Product5/2
  vel/1 -> Demux/1
  inertia(3x3)/1 -> Product1/2
  "mass(3x3) "/1 -> Mux/1
  Sum/1 -> Mux/2
  Mux/1 -> force/1

== system P_decouple_cascade_rov/inner-loop controller/inner -backstepping/M+Ma_pert ==
  selector : Inport  Port=1  LatchInput=off
  Mux : Mux  Inputs=6
  Mux1 : Mux  Inputs=6
  Subsystem : Subsystem
  Subsystem1 : Subsystem
  Subsystem2 : Subsystem
  Subsystem3 : Subsystem
  Subsystem4 : Subsystem
  Subsystem5 : Subsystem
  M+Ma_pert : Outport
  "M " : Outport  Port=2
  wires:
  Subsystem/1(M+Ma (1,1)) -> Mux/1
  selector/1 -> Subsystem/1(M_select), Subsystem1/1(M_select), Subsystem2/1(M_select), Subsystem3/1(M_select), Subsystem4/1(M_select), Subsystem5/1(M_select)
  Subsystem1/1(M+Ma (2,2)) -> Mux/2
  Subsystem2/1(M+Ma (3,3)) -> Mux/3
  Subsystem3/1(M+Ma (4,4)) -> Mux/4
  Subsystem4/1(M+Ma (5,5)) -> Mux/5
  Subsystem5/1(M+Ma (6,6)) -> Mux/6
  Subsystem/2("M (1,1) ") -> Mux1/1
  Subsystem1/2("M (2,2) ") -> Mux1/2
  Subsystem2/2("M (3,3) ") -> Mux1/3
  Subsystem3/2("M (4,4) ") -> Mux1/4
  Subsystem4/2("M (5,5) ") -> Mux1/5
  Subsystem5/2("M (6,6) ") -> Mux1/6
  Mux/1 -> M+Ma_pert/1
  Mux1/1 -> "M "/1

== system P_decouple_cascade_rov/inner-loop controller/inner -backstepping/backstepping-x ==
  M+Ma_pert-x : Inport  Orientation=down  Port=1  LatchInput=off
  C+Ca+C_pert-y : Inport  Port=2  LatchInput=off
  err : Inport  Port=3  LatchInput=off
  1+(Yvdot+d_Yvdot)vr : Sum  Inputs=|++  SaturateOnIntegerOverflow=on  InputSameDT=on
  1+(Yvdot+d_Yvdot)vr1 : Sum  Inputs=|+-++  SaturateOnIntegerOverflow=on  InputSameDT=on
  Constant : Constant
  "Ku " : Constant  Value=21
  Ku1 : Gain  Gain=2
  Math Function : Math  Operator=reciprocal  SaturateOnIntegerOverflow=on
  Math Function1 : Math  Operator=square  SaturateOnIntegerOverflow=on
  Selector : Selector  Elements=[1]  InputPortWidth=6
  vp*rp2 : Product  Inputs=4  SaturateOnIntegerOverflow=on  RndMeth=Zero  InputSameDT=on
  ubar_ix : Outport
  wires:
  Constant/1 -> 1+(Yvdot+d_Yvdot)vr/1, 1+(Yvdot+d_Yvdot)vr1/4
  Math Function/1 -> vp*rp2/1
  1+(Yvdot+d_Yvdot)vr/1 -> vp*rp2/2
  1+(Yvdot+d_Yvdot)vr1/1 -> Math Function/1
  M+Ma_pert-x/1 -> vp*rp2/3, 1+(Yvdot+d_Yvdot)vr1/3
  "Ku "/1 -> Ku1/1, Math Function1/1
  Ku1/1 -> 1+(Yvdot+d_Yvdot)vr1/2
  Math Function1/1 -> 1+(Yvdot+d_Yvdot)vr1/1
  vp*rp2/1 -> ubar_ix/1
  C+Ca+C_pert-y/1 -> 1+(Yvdot+d_Yvdot)vr/2
  err/1 -> Selector/1
  Selector/1 -> vp*rp2/4

== system P_decouple_cascade_rov/inner-loop controller/inner -backstepping/backstepping-y ==
  M+Ma_pert-y : Inport  Orientation=down  Port=1  LatchInput=off
  m : Inport  Port=2  LatchInput=off
  "err  " : Inport  Port=3  LatchInput=off
  1+(Yvdot+d_Yvdot)vr1 : Sum  Inputs=|+-++  SaturateOnIntegerOverflow=on  InputSameDT=on
  1+mur : Sum  Inputs=|++  SaturateOnIntegerOverflow=on  InputSameDT=on
  Constant : Constant
  Demux3 : Demux  Outputs=6
  Ku1 : Gain  Gain=2
  "Kv " : Constant  Value=22
  Math Function : Math  Operator=reciprocal  SaturateOnIntegerOverflow=on
  Math Function1 : Math  Operator=square  SaturateOnIntegerOverflow=on
  vp*rp1 : Product  Inputs=3  SaturateOnIntegerOverflow=on  RndMeth=Zero  InputSameDT=on
  vp*rp2 : Product  Inputs=4  SaturateOnIntegerOverflow=on  RndMeth=Zero  InputSameDT=on
  ubar_iy : Outport
  wires:
  Constant/1 -> 1+mur/1, 1+(Yvdot+d_Yvdot)vr1/4
  Math Function/1 -> vp*rp2/1
  1+mur/1 -> vp*rp2/2
  1+(Yvdot+d_Yvdot)vr1/1 -> Math Function/1
  M+Ma_pert-y/1 -> vp*rp2/3, 1+(Yvdot+d_Yvdot)vr1/3
  "Kv "/1 -> Ku1/1, Math Function1/1
  Ku1/1 -> 1+(Yvdot+d_Yvdot)vr1/2
  Math Function1/1 -> 1+(Yvdot+d_Yvdot)vr1/1
  vp*rp2/1 -> ubar_iy/1
  vp*rp1/1 -> 1+mur/2
  m/1 -> vp*rp1/1
  Demux3/6 -> vp*rp1/3
  Demux3/2 -> vp*rp2/4
  "err  "/1 -> Demux3/1
  Demux3/1 -> vp*rp1/2

== system P_decouple_cascade_rov/inner-loop controller/inner -backstepping/backstepping-yaw ==
  M+Ma_pert-yaw : Inport  Orientation=down  Port=1  LatchInput=off
  C+Ca+C_pert-x : Inport  Port=2  LatchInput=off
  err : Inport  Port=3  LatchInput=off
  1+(Xudot+d_Xudot)uv : Sum  Inputs=|++  SaturateOnIntegerOverflow=on  InputSameDT=on
  1+(Yvdot+d_Yvdot)vr1 : Sum  Inputs=|+-++  SaturateOnIntegerOverflow=on  InputSameDT=on
  Constant : Constant
  "Kr " : Constant  Value=22
  Ku1 : Gain  Gain=2
  Math Function : Math  Operator=reciprocal  SaturateOnIntegerOverflow=on
  Math Function1 : Math  Operator=square  SaturateOnIntegerOverflow=on
  Selector : Selector  Elements=[6]  InputPortWidth=6
  vp*rp2 : Product  Inputs=4  SaturateOnIntegerOverflow=on  RndMeth=Zero  InputSameDT=on
  ubar_iyaw : Outport
  wires:
  Constant/1 -> 1+(Xudot+d_Xudot)uv/1, 1+(Yvdot+d_Yvdot)vr1/4
  Math Function/1 -> vp*rp2/1
  1+(Xudot+d_Xudot)uv/1 -> vp*rp2/2
  1+(Yvdot+d_Yvdot)vr1/1 -> Math Function/1
  M+Ma_pert-yaw/1 -> vp*rp2/3, 1+(Yvdot+d_Yvdot)vr1/3
  "Kr "/1 -> Ku1/1, Math Function1/1
  Ku1/1 -> 1+(Yvdot+d_Yvdot)vr1/2
  Math Function1/1 -> 1+(Yvdot+d_Yvdot)vr1/1
  vp*rp2/1 -> ubar_iyaw/1
  C+Ca+C_pert-x/1 -> 1+(Xudot+d_Xudot)uv/2
  err/1 -> Selector/1
  Selector/1 -> vp*rp2/4

== system P_decouple_cascade_rov/inner-loop controller/inner -backstepping/backstepping-z ==
  M+Ma_pert-z : Inport  Orientation=down  Port=1  LatchInput=off
  "err  " : Inport  Port=2  LatchInput=off
  1+(Yvdot+d_Yvdot)vr1 : Sum  Inputs=|+-++  SaturateOnIntegerOverflow=on  InputSameDT=on
  Constant : Constant
  Ku1 : Gain  Gain=2
  "Kw " : Constant  Value=23
  Math Function : Math  Operator=reciprocal  SaturateOnIntegerOverflow=on
  Math Function1 : Math  Operator=square  SaturateOnIntegerOverflow=on
  Selector : Selector  Elements=[3]  InputPortWidth=6
  vp*rp2 : Product  Inputs=3  SaturateOnIntegerOverflow=on  RndMeth=Zero  InputSameDT=on
  ubar_iz : Outport
  wires:
  Constant/1 -> 1+(Yvdot+d_Yvdot)vr1/4
  Math Function/1 -> vp*rp2/1
  1+(Yvdot+d_Yvdot)vr1/1 -> Math Function/1
  M+Ma_pert-z/1 -> 1+(Yvdot+d_Yvdot)vr1/3, vp*rp2/2
  "Kw "/1 -> Ku1/1, Math Function1/1
  Ku1/1 -> 1+(Yvdot+d_Yvdot)vr1/2
  Math Function1/1 -> 1+(Yvdot+d_Yvdot)vr1/1
  vp*rp2/1 -> ubar_iz/1
  "err  "/1 -> Selector/1
  Selector/1 -> vp*rp2/3

== system P_decouple_cascade_rov/inner-loop controller/inner -backstepping/thruster  dynamic     1 ==
  volt : Inport  Orientation=down  Port=1  LatchInput=off
  Gain2 : Gain  Gain=0.5  SaturateOnIntegerOverflow=on
  Saturation : Saturate  UpperLimit=70  LowerLimit=-70
  "thruster  alloc. " : Subsystem
  T : Outport
  wires:
  volt/1 -> "thruster  alloc. "/1(err)
  "thruster  alloc. "/1(u) -> Gain2/1
  Saturation/1 -> T/1
  Gain2/1 -> Saturation/1

== system P_decouple_cascade_rov/inner-loop controller/inner -backstepping/upper limit (diag)    ==
  note: 7 8 9 10 11 12
  note: 1 2 3 4 5 6
  vel : Inport  Port=1  LatchInput=off
  (zg.W - zb.B)cY.sX : Fcn  Expr=-u[9]*u[3]*u[5]+u[8]*u[2]*u[6]
  (zg.W - zb.B)cY.sX1 : Fcn  Expr=u[9]*u[3]*u[4]-u[7]*u[1]*u[6]
  (zg.W - zb.B)cY.sX2 : Fcn  Expr=-u[8]*u[2]*u[4]+u[7]*u[1]*u[5]
  (zg.W - zb.B)cY.sX3 : Fcn  Expr=-u[9]*u[3]*u[2]+u[8]*u[2]*u[3]-u[12]*u[6]*u[5]+u[11]*u[5]*u[6]
  (zg.W - zb.B)cY.sX4 : Fcn  Expr=u[9]*u[3]*u[1]-u[7]*u[1]*u[3]+u[6]*u[12]*u[4]-u[4]*u[10]*u[6]
  (zg.W - zb.B)cY.sX5 : Fcn  Expr=-u[8]*u[2]*u[1]+u[7]*u[1]*u[2]-u[11]*u[5]*u[4]+u[10]*u[4]*u[5]
  Mux1 : Mux  Inputs=6
  Mux3 : Mux  Inputs=2
  Rg2 : Constant  Value="[MaU(1)  MaU(2)  MaU(3)  MaU(4)  MaU(5)  MaU(6) ]'"
  force : Outport
  wires:
  Mux1/1 -> force/1
  (zg.W - zb.B)cY.sX/1 -> Mux1/1
  (zg.W - zb.B)cY.sX1/1 -> Mux1/2
  (zg.W - zb.B)cY.sX2/1 -> Mux1/3
  (zg.W - zb.B)cY.sX3/1 -> Mux1/4
  (zg.W - zb.B)cY.sX4/1 -> Mux1/5
  (zg.W - zb.B)cY.sX5/1 -> Mux1/6
  vel/1 -> Mux3/1
  Rg2/1 -> Mux3/2
  Mux3/1 -> (zg.W - zb.B)cY.sX/1, (zg.W - zb.B)cY.sX1/1, (zg.W - zb.B)cY.sX4/1, (zg.W - zb.B)cY.sX5/1, (zg.W - zb.B)cY.sX3/1, (zg.W - zb.B)cY.sX2/1

== system P_decouple_cascade_rov/inner-loop controller/inner -backstepping/upper limit (diag)   1 ==
  note: 7 8 9 10 11 12
  note: 1 2 3 4 5 6
  vel : Inport  Port=1  LatchInput=off
  (zg.W - zb.B)cY.sX : Fcn  Expr=-u[9]*u[3]*u[5]+u[8]*u[2]*u[6]
  (zg.W - zb.B)cY.sX1 : Fcn  Expr=u[9]*u[3]*u[4]-u[7]*u[1]*u[6]
  (zg.W - zb.B)cY.sX2 : Fcn  Expr=-u[8]*u[2]*u[4]+u[7]*u[1]*u[5]
  (zg.W - zb.B)cY.sX3 : Fcn  Expr=-u[9]*u[3]*u[2]+u[8]*u[2]*u[3]-u[12]*u[6]*u[5]+u[11]*u[5]*u[6]
  (zg.W - zb.B)cY.sX4 : Fcn  Expr=u[9]*u[3]*u[1]-u[7]*u[1]*u[3]+u[6]*u[12]*u[4]-u[4]*u[10]*u[6]
  (zg.W - zb.B)cY.sX5 : Fcn  Expr=-u[8]*u[2]*u[1]+u[7]*u[1]*u[2]-u[11]*u[5]*u[4]+u[10]*u[4]*u[5]
  Mux1 : Mux  Inputs=6
  Mux3 : Mux  Inputs=2
  Rg1 : Constant  Value="[Ma(1)  Ma(2)  Ma(3)  Ma(4)  Ma(5)  Ma(6) ]'"
  force : Outport
  wires:
  Mux1/1 -> force/1
  (zg.W - zb.B)cY.sX/1 -> Mux1/1
  (zg.W - zb.B)cY.sX1/1 -> Mux1/2
  (zg.W - zb.B)cY.sX2/1 -> Mux1/3
  (zg.W - zb.B)cY.sX3/1 -> Mux1/4
  (zg.W - zb.B)cY.sX4/1 -> Mux1/5
  (zg.W - zb.B)cY.sX5/1 -> Mux1/6
  vel/1 -> Mux3/1
  Rg1/1 -> Mux3/2
  Mux3/1 -> (zg.W - zb.B)cY.sX/1, (zg.W - zb.B)cY.sX1/1, (zg.W - zb.B)cY.sX4/1, (zg.W - zb.B)cY.sX5/1, (zg.W - zb.B)cY.sX3/1, (zg.W - zb.B)cY.sX2/1

== system P_decouple_cascade_rov/inner-loop controller/inner-P/thruster  dynamic     1 ==
  volt : Inport  Orientation=down  Port=1  LatchInput=off
  Gain2 : Gain  Gain=0.5  SaturateOnIntegerOverflow=on
  Saturation : Saturate  UpperLimit=70  LowerLimit=-70
  "thruster  alloc. " : Subsystem
  T : Outport
  wires:
  volt/1 -> "thruster  alloc. "/1(err)
  "thruster  alloc. "/1(u) -> Gain2/1
  Saturation/1 -> T/1
  Gain2/1 -> Saturation/1

== system P_decouple_cascade_rov/inner-loop controller/inner-sliding/thruster  dynamic     1 ==
  volt : Inport  Orientation=down  Port=1  LatchInput=off
  Gain2 : Gain  Gain=0.5  SaturateOnIntegerOverflow=on
  Saturation : Saturate  UpperLimit=70  LowerLimit=-70
  "thruster  alloc. " : Subsystem
  T : Outport
  wires:
  volt/1 -> "thruster  alloc. "/1(err)
  "thruster  alloc. "/1(u) -> Gain2/1
  Saturation/1 -> T/1
  Gain2/1 -> Saturation/1
